simulink model "part4_2state_simulation"  (R2014a)
settings: Solver=ode45  StartTime=0.0  StopTime=10  MaxStep=.001  RelTol=1e-3
settings Model: Creator=nandi2  LastModifiedBy=nandi2

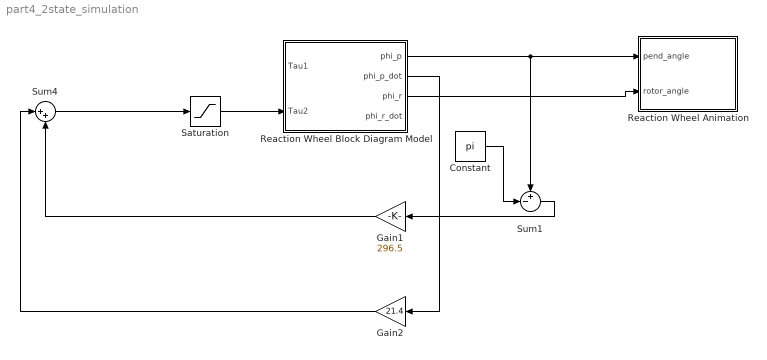
== system part4_2state_simulation ==
  Constant : Constant  Value=pi
  Gain1 : Gain  Gain=296.5
  Gain2 : Gain  Gain=21.4
  Reaction Wheel Animation : Subsystem  mask(Reaction Wheel Animation){}
      mask help: The animation block takes as input the pendulum angle (in radians), with 0 pointing down. Use this to visualize the pendulum position while testing controllers.
      mask Help: The animation block takes as input the pendulum angle (in radians), with 0 pointing down.  Use this to visualize the pendulum position while testing controllers.
      mask Display:
      | port_label('input', 1, 'phi_p')
      | port_label('input', 2, 'phi_r')
      | fprintf('RWP Animation')
  Reaction Wheel Block Diagram Model : Subsystem  mask(Reaction Wheel Block Diagram Model){par=[69.25 .935 178], g=9.804, init=[pi 0 0 0]}
      mask prompts: par "Internal Parameters (a, bp, br)"; g "Acceleration of Gravity"; init "Initial Conditions"
      mask help:
      | This is a <i>nonlinear mathematical model</i> of the reaction wheel pendulum.  It takes as inputs torques to the system, and outputs a state vector.
      | <p>
      | <h2>Parameters</h2>
      | <ul>
      | <h3>Internal Parameters</h3>
      | <ul>
      | <li><b>a</b>, the square of the frquency of small oscillations ( a = omega<sub>p</sub><sup>2</sup>) </li>
      | <li><b>b<sub>p</sub></b>, the control gain over total inertia (b<sub>p</sub> = k<sub>u</sub>/J)</li>
      | <li><b>b<sub>r</sub></b>, the control gain over rotor inertia (b<sub>r</sub> = k<sub>u</sub>/J<sub>r</sub>)</li>
      | </ul>
      | <h3>Acceleration of Gravity</h3>
      | <ul>
      | <li><b>g</b>, commonly 9.804</li>
      | </ul>
      | <h3>Initial Conditions</h3>
      | Starting values for the state vector.  Usually, use [pi, 0,0,0] to start the pendulum at rest in the unstable equilibrium position pointing upwards.
      | <ul>
      | <li><b>phi<sub>p</sub></b>, encoder angle of the pendulum, in radians (0 is down)</li>
      | <li><b>phi<sub>p</sub>dot</b>, angular velocity of the pendulum, in radians/sec</li>
      | <li><b>phi<sub>r</sub></b>, encoder angle of the rotor, in radians (0 is down)</li>
      | <li><b>phi<sub>r</sub>dot</b>, angular velocity of the pendulum, in radians/sec</li>
      | </ul>
      | </ul>
      | <p>
      mask Help:
      | This is a <i>nonlinear mathematical model</i>  of the reaction wheel pendulum.  It takes as inputs torques to the system, and outputs a state vector.
      | <p>
      | <h2>Parameters</h2>
      | <ul>
      | <h3>Internal Parameters</h3>
      | <ul>
      | <li><b>a</b>, the square of the frquency of small oscillations ( a = omega<sub>p</sub><sup>2</sup>) </li>
      | <li><b>b<sub>p</sub></b>, the control gain over total inertia (b<sub>p</sub> = k<sub>u</sub>/J)</li>
      | <li><b>b<sub>r</sub></b>, the control gain over rotor inertia (b<sub>r</sub> = k<sub>u</sub>/J<sub>r</sub>)</li>
      | </ul>
      | <h3>Acceleration of Gravity</h3>
      | <ul>
      | <li><b>g</b>, commonly 9.804</li>
      | </ul>
      | <h3>Initial Conditions</h3>
      | Starting values for the state vector.  Usually, use [pi, 0,0,0] to start the pendulum at rest in the unstable equilibrium position pointing upwards.
      | <ul>
      | <li><b>phi<sub>p</sub></b>, encoder angle of the pendulum, in radians (0 is down)</li>
      | <li><b>phi<sub>p</sub>dot</b>, angular velocity of the pendulum, in radians/sec</li>
      | <li><b>phi<sub>r</sub></b>, encoder angle of the rotor, in radians (0 is down)</li>
      | <li><b>phi<sub>r</sub>dot</b>, angular velocity of the pendulum, in radians/sec</li>
      | </ul>
      | </ul>
      | <p>
      | 
      | <h2>Inputs</h2>
      | <ul>
      | <li><b>Tau1</b>, external force on the pendulum arm. (This arm is not actuated, but disturbances can be applied here)</li>
      | <li><b>Tau2</b>, external force on the rotor.  (input to the motor + disturbances)</li>
      | </ul>
      | 
      | <h2>Outputs</h2>
      | <ul>
      |  Outputs the current state vector. (See Initial Conditions)
      | </ul>
      | <p>
      | Don’t forget to include a Saturation block (to saturate the control effort at +/- 10) before <i>Tau2</i>.
      | <p>
      | <!-- last updates, Summer, 2007 -->
  Saturation : Saturate  UpperLimit=10  LowerLimit=-10
  Sum1 : Sum  Inputs=+-|
  Sum4 : Sum  Inputs=|++
  wires:
  Reaction Wheel Block Diagram Model/1(phi_p) -> Sum1/1, Reaction Wheel Animation/1(pend_angle)
  Reaction Wheel Block Diagram Model/3(phi_r) -> Reaction Wheel Animation/2(rotor_angle)
  Gain1/1 -> Sum4/2
  Gain2/1 -> Sum4/1
  Sum4/1 -> Saturation/1
  Saturation/1 -> Reaction Wheel Block Diagram Model/2(Tau2)
  Reaction Wheel Block Diagram Model/2(phi_p_dot) -> Gain2/1
  Constant/1 -> Sum1/2
  Sum1/1 -> Gain1/1

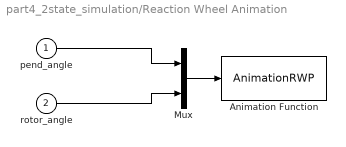
== system part4_2state_simulation/Reaction Wheel Animation ==
  pend_angle : Inport
  rotor_angle : Inport  Port=2
  Animation Function : S-Function  FunctionName=AnimationRWP  Parameters=0.05  EnableBusSupport=off
      settings: DeleteFcn=if ~isempty(findobj('type','figure','name','dblpend1 Animation'));close('dblpend1 Animation'); end;
  Mux : Mux  Inputs=2
  wires:
  pend_angle/1 -> Mux/1
  rotor_angle/1 -> Mux/2
  Mux/1 -> Animation Function/1

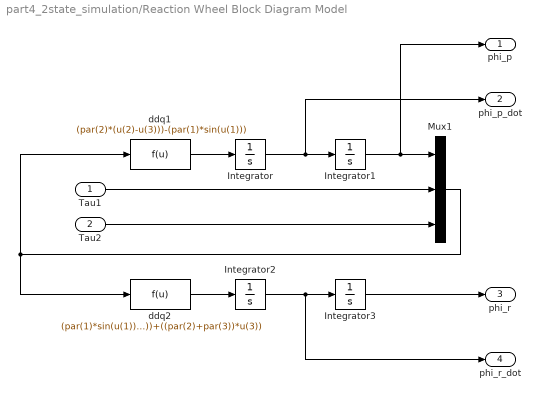
== system part4_2state_simulation/Reaction Wheel Block Diagram Model ==
  Tau1 : Inport
  Tau2 : Inport  Port=2
  Integrator : Integrator  InitialCondition=init(2)
  Integrator1 : Integrator  InitialCondition=init(1)
  Integrator2 : Integrator  InitialCondition=init(4)
  Integrator3 : Integrator  InitialCondition=init(3)
  Mux1 : Mux  Inputs=3
  ddq1 : Fcn  Expr=(par(2)*(u(2)-u(3)))-(par(1)*sin(u(1)))
  ddq2 : Fcn  Expr=(par(1)*sin(u(1)))-(par(2)*u(2))+((par(2)+par(3))*u(3))
  phi_p : Outport
  phi_p_dot : Outport  Port=2
  phi_r : Outport  Port=3
  phi_r_dot : Outport  Port=4
  wires:
  ddq1/1 -> Integrator/1
  ddq2/1 -> Integrator2/1
  Integrator3/1 -> phi_r/1
  Integrator2/1 -> phi_r_dot/1, Integrator3/1
  Integrator/1 -> phi_p_dot/1, Integrator1/1
  Integrator1/1 -> phi_p/1, Mux1/1
  Tau1/1 -> Mux1/2
  Tau2/1 -> Mux1/3
  Mux1/1 -> ddq2/1, ddq1/1
